simulink model "classical_modern_interplay"  (R2022b)
settings: Solver=VariableStepAuto  StartTime=0.0  StopTime=20  MaxStep=.05  RelTol=1e-3
values from neighbouring files (symbols this model uses):
  k1 = .46    (= 0.46)    [partial_state_feedback.m]
  k2 = .68    (= 0.68)    [partial_state_feedback.m]
  sys_ss = ss([0 1;-1 -1], [0;1], [1 0], 0)    [partial_state_feedback.m]
undefined symbols (not defined in the file or in its folder): k3
settings Model: Creator=hp_desktop  LastModifiedBy=hp_desktop

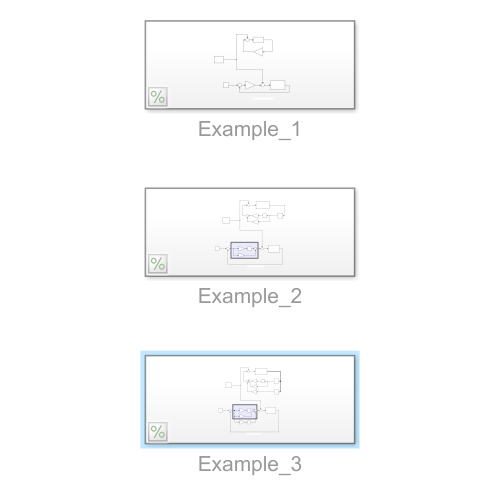
[thumbnail: Simulink's stored preview of the top-level diagram]
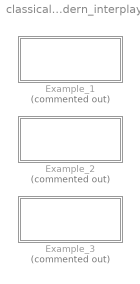
== system classical_modern_interplay ==
  Example_1 : Subsystem  Commented=on
  Example_2 : Subsystem  Commented=on
  Example_3 : Subsystem  Commented=on

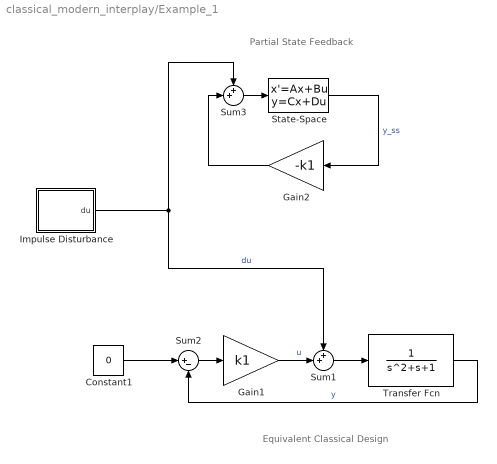
== system classical_modern_interplay/Example_1 ==
  note: Partial State Feedback
  note: Equivalent Classical Design
  Constant1 : Constant  Value=0
  Gain1 : Gain  Gain=k1
  Gain2 : Gain  Gain=-k1
  Impulse Disturbance : Subsystem
  State-Space : StateSpace  A=sys_ss.A  B=sys_ss.B  C=sys_ss.C  D=sys_ss.D  InitialCondition=[0;0]
  Sum1 : Sum  Inputs=++|
  Sum2 : Sum  Inputs=|+-
  Sum3 : Sum  Inputs=++|
  Transfer Fcn : TransferFcn  Denominator=[1 1 1]
  wires:
  Sum2/1 -> Gain1/1
  Sum3/1 -> State-Space/1
  Constant1/1 -> Sum2/1
  State-Space/1 -> Gain2/1  "y_ss"
  Transfer Fcn/1 -> Sum2/2  "y"
  Gain2/1 -> Sum3/2
  Sum1/1 -> Transfer Fcn/1
  Gain1/1 -> Sum1/2  "u"
  Impulse Disturbance/1(du) -> Sum3/1, Sum1/1  "du"

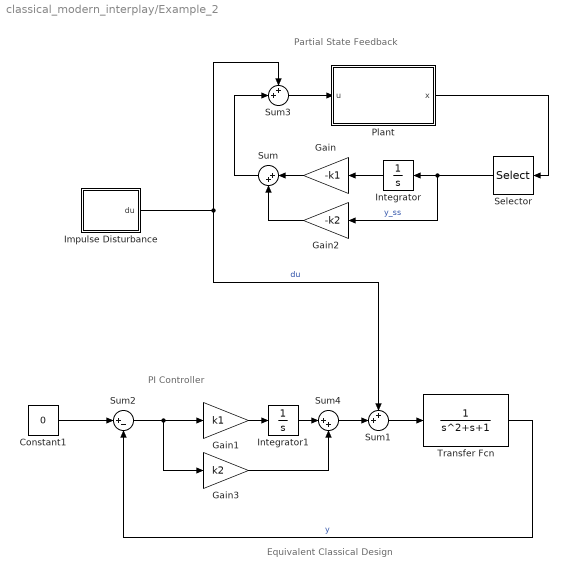
== system classical_modern_interplay/Example_2 ==
  note: PI Controller
  note: Equivalent Classical Design
  note: Partial State Feedback
  Constant1 : Constant  Value=0
  Gain : Gain  Gain=-k1
  Gain1 : Gain  Gain=k1
  Gain2 : Gain  Gain=-k2
  Gain3 : Gain  Gain=k2
  Impulse Disturbance : Subsystem
  Integrator : Integrator
  Integrator1 : Integrator
  Plant : Subsystem
  Selector : Selector  InputPortWidth=2  IndexOptions=Index vector (dialog)  Indices=1  OutputSizes=1
  Sum : Sum  Inputs=|++
  Sum1 : Sum  Inputs=++|
  Sum2 : Sum  Inputs=|+-
  Sum3 : Sum  Inputs=++|
  Sum4 : Sum  Inputs=|++
  Transfer Fcn : TransferFcn  Denominator=[1 1 1]
  wires:
  Impulse Disturbance/1(du) -> Sum1/1, Sum3/1  "du"
  Sum1/1 -> Transfer Fcn/1
  Transfer Fcn/1 -> Sum2/2  "y"
  Constant1/1 -> Sum2/1
  Sum3/1 -> Plant/1(u)
  Plant/1(x) -> Selector/1
  Selector/1 -> Gain2/1, Integrator/1  "y_ss"
  Gain/1 -> Sum/1
  Integrator/1 -> Gain/1
  Gain2/1 -> Sum/2
  Sum/1 -> Sum3/2
  Gain1/1 -> Integrator1/1
  Integrator1/1 -> Sum4/1
  Gain3/1 -> Sum4/2
  Sum4/1 -> Sum1/2
  Sum2/1 -> Gain3/1, Gain1/1

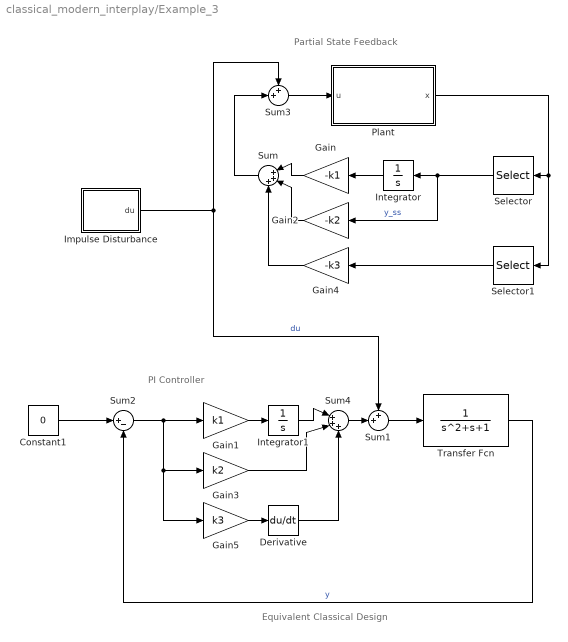
== system classical_modern_interplay/Example_3 ==
  note: Partial State Feedback
  note: Equivalent Classical Design
  note: PI Controller
  Constant1 : Constant  Value=0
  Derivative : Derivative
  Gain : Gain  Gain=-k1
  Gain1 : Gain  Gain=k1
  Gain2 : Gain  Gain=-k2
  Gain3 : Gain  Gain=k2
  Gain4 : Gain  Gain=-k3
  Gain5 : Gain  Gain=k3
  Impulse Disturbance : Subsystem
  Integrator : Integrator
  Integrator1 : Integrator
  Plant : Subsystem
  Selector : Selector  InputPortWidth=2  IndexOptions=Index vector (dialog)  Indices=1  OutputSizes=1
  Selector1 : Selector  InputPortWidth=2  IndexOptions=Index vector (dialog)  Indices=2  OutputSizes=1
  Sum : Sum  Inputs=|+++
  Sum1 : Sum  Inputs=++|
  Sum2 : Sum  Inputs=|+-
  Sum3 : Sum  Inputs=++|
  Sum4 : Sum  Inputs=|+++
  Transfer Fcn : TransferFcn  Denominator=[1 1 1]
  wires:
  Sum2/1 -> Gain1/1, Gain5/1, Gain3/1
  Sum4/1 -> Sum1/2
  Gain3/1 -> Sum4/2
  Integrator1/1 -> Sum4/1
  Gain1/1 -> Integrator1/1
  Sum/1 -> Sum3/2
  Gain2/1 -> Sum/2
  Integrator/1 -> Gain/1
  Gain/1 -> Sum/1
  Selector/1 -> Integrator/1, Gain2/1  "y_ss"
  Plant/1(x) -> Selector1/1, Selector/1
  Sum3/1 -> Plant/1(u)
  Constant1/1 -> Sum2/1
  Transfer Fcn/1 -> Sum2/2  "y"
  Sum1/1 -> Transfer Fcn/1
  Impulse Disturbance/1(du) -> Sum3/1, Sum1/1  "du"
  Selector1/1 -> Gain4/1
  Gain4/1 -> Sum/3
  Gain5/1 -> Derivative/1
  Derivative/1 -> Sum4/3

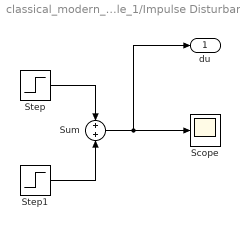
== system classical_modern_interplay/Example_1/Impulse Disturbance ==
  Scope : Scope
  Step : Step  Time=3  SampleTime=0
  Step1 : Step  Time=3.2  After=-1  SampleTime=0
  Sum : Sum
  du : Outport
  wires:
  Sum/1 -> du/1, Scope/1
  Step/1 -> Sum/1
  Step1/1 -> Sum/2

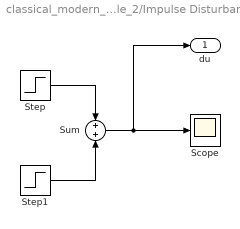
== system classical_modern_interplay/Example_2/Impulse Disturbance ==
  Scope : Scope
  Step : Step  Time=3  SampleTime=0
  Step1 : Step  Time=3.2  After=-1  SampleTime=0
  Sum : Sum
  du : Outport
  wires:
  Step1/1 -> Sum/2
  Step/1 -> Sum/1
  Sum/1 -> Scope/1, du/1

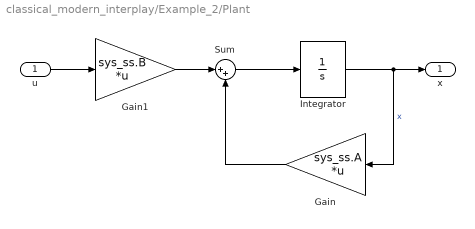
== system classical_modern_interplay/Example_2/Plant ==
  u : Inport
  Gain : Gain  Gain=sys_ss.A  Multiplication=Matrix(K*u)
  Gain1 : Gain  Gain=sys_ss.B  Multiplication=Matrix(K*u)
  Integrator : Integrator  InitialCondition=[0;0]
  Sum : Sum  Inputs=|++
  x : Outport
  wires:
  Integrator/1 -> x/1, Gain/1  "x"
  u/1 -> Gain1/1
  Gain/1 -> Sum/2
  Sum/1 -> Integrator/1
  Gain1/1 -> Sum/1

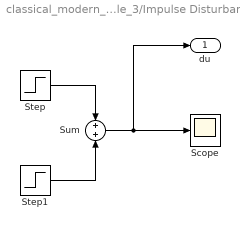
== system classical_modern_interplay/Example_3/Impulse Disturbance ==
  Scope : Scope
  Step : Step  Time=3  SampleTime=0
  Step1 : Step  Time=3.2  After=-1  SampleTime=0
  Sum : Sum
  du : Outport
  wires:
  Sum/1 -> du/1, Scope/1
  Step/1 -> Sum/1
  Step1/1 -> Sum/2

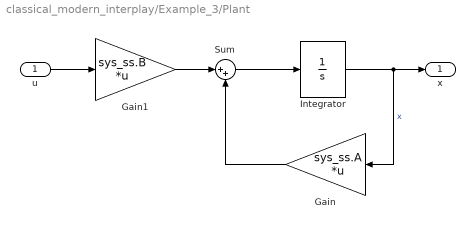
== system classical_modern_interplay/Example_3/Plant ==
  u : Inport
  Gain : Gain  Gain=sys_ss.A  Multiplication=Matrix(K*u)
  Gain1 : Gain  Gain=sys_ss.B  Multiplication=Matrix(K*u)
  Integrator : Integrator  InitialCondition=[0;0]
  Sum : Sum  Inputs=|++
  x : Outport
  wires:
  Gain1/1 -> Sum/1
  Sum/1 -> Integrator/1
  Gain/1 -> Sum/2
  u/1 -> Gain1/1
  Integrator/1 -> Gain/1, x/1  "x"
